simulink model "CoP"  (R2014a)
settings: Solver=ode45  StartTime=0.0  StopTime=10.0  RelTol=1e-3
values from neighbouring files (symbols this model uses):
  l_ankle_pitch = 18    [parameters.m]
  l_ankle_roll = 19    [parameters.m]
libraries: WBCLibrary x6
settings Model: Creator=luca  LastModifiedBy=luca

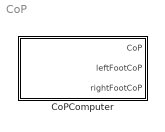
== system CoP ==
  CoPComputer : Subsystem

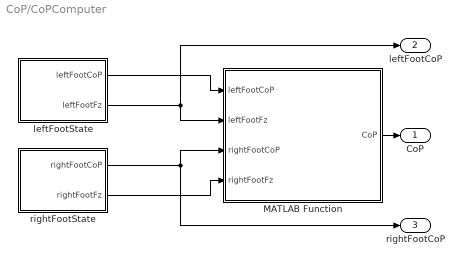
== system CoP/CoPComputer ==
  MATLAB Function : MATLAB Function  TreatAsAtomicUnit=on
  leftFootState : Subsystem
  rightFootState : Subsystem
  CoP : Outport
  leftFootCoP : Outport  Port=2
  rightFootCoP : Outport  Port=3
  wires:
  rightFootState/1(rightFootCoP) -> rightFootCoP/1, MATLAB Function/3(rightFootCoP)
  leftFootState/1(leftFootCoP) -> MATLAB Function/1(leftFootCoP)
  leftFootState/2(leftFootFz) -> leftFootCoP/1, MATLAB Function/2(leftFootFz)
  rightFootState/2(rightFootFz) -> MATLAB Function/4(rightFootFz)
  MATLAB Function/1(CoP) -> CoP/1

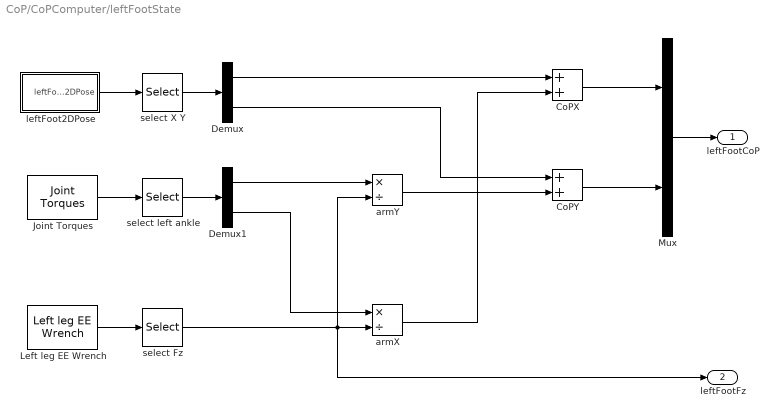
== system CoP/CoPComputer/leftFootState ==
  CoPX : Sum
  CoPY : Sum
  Demux : Demux  Outputs=2
  Demux1 : Demux  Outputs=2
  Joint Torques : WBCLibrary/wholeBodyStates/Joint Torques  robotName=robotName  localName=localName
  Left leg EE Wrench : WBCLibrary/wholeBodyStates/Left leg EE Wrench  robotName=robotName  localName=localName
  Mux : Mux  Inputs=2
  armX : Product  Inputs=*/
  armY : Product  Inputs=*/
  leftFoot2DPose : Subsystem
  select Fz : Selector  InputPortWidth=25  Indices=[3]
  select X Y : Selector  InputPortWidth=25  Indices=[1, 2]
  select left ankle : Selector  InputPortWidth=25  Indices=[l_ankle_pitch, l_ankle_roll]
  leftFootCoP : Outport
  leftFootFz : Outport  Port=2
  wires:
  Left leg EE Wrench/1 -> select Fz/1
  select left ankle/1 -> Demux1/1
  CoPY/1 -> Mux/2
  CoPX/1 -> Mux/1
  armY/1 -> CoPY/2
  Mux/1 -> leftFootCoP/1
  Demux1/2 -> armX/1
  Demux/2 -> CoPY/1
  Demux/1 -> CoPX/1
  Joint Torques/1 -> select left ankle/1
  armX/1 -> CoPX/2
  Demux1/1 -> armY/1
  select X Y/1 -> Demux/1
  leftFoot2DPose/1(leftFoot2DPose) -> select X Y/1
  select Fz/1 -> leftFootFz/1, armX/2, armY/2

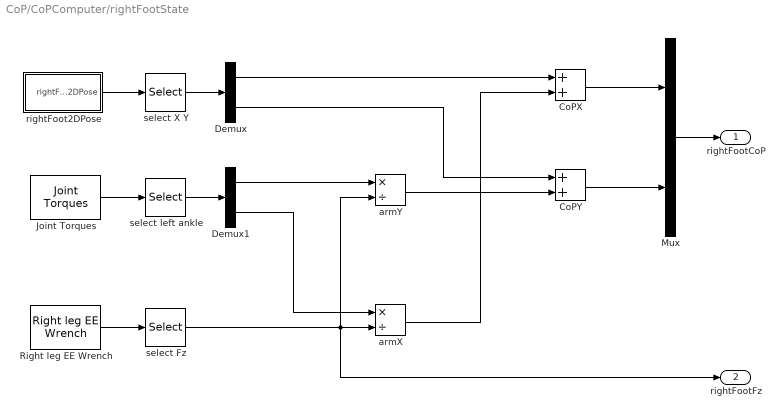
== system CoP/CoPComputer/rightFootState ==
  CoPX : Sum
  CoPY : Sum
  Demux : Demux  Outputs=2
  Demux1 : Demux  Outputs=2
  Joint Torques : WBCLibrary/wholeBodyStates/Joint Torques  robotName=robotName  localName=localName
  Mux : Mux  Inputs=2
  Right leg EE Wrench : WBCLibrary/wholeBodyStates/Right leg EE Wrench  robotName=robotName  localName=localName
  armX : Product  Inputs=*/
  armY : Product  Inputs=*/
  rightFoot2DPose : Subsystem
  select Fz : Selector  InputPortWidth=25  Indices=[3]
  select X Y : Selector  InputPortWidth=25  Indices=[1, 2]
  select left ankle : Selector  InputPortWidth=25  Indices=[l_ankle_pitch, l_ankle_roll]
  rightFootCoP : Outport
  rightFootFz : Outport  Port=2
  wires:
  Right leg EE Wrench/1 -> select Fz/1
  select left ankle/1 -> Demux1/1
  CoPY/1 -> Mux/2
  CoPX/1 -> Mux/1
  armY/1 -> CoPY/2
  Mux/1 -> rightFootCoP/1
  Demux1/2 -> armX/1
  Demux/2 -> CoPY/1
  Demux/1 -> CoPX/1
  Joint Torques/1 -> select left ankle/1
  armX/1 -> CoPX/2
  Demux1/1 -> armY/1
  select X Y/1 -> Demux/1
  rightFoot2DPose/1(rightFoot2DPose) -> select X Y/1
  select Fz/1 -> rightFootFz/1, armX/2, armY/2

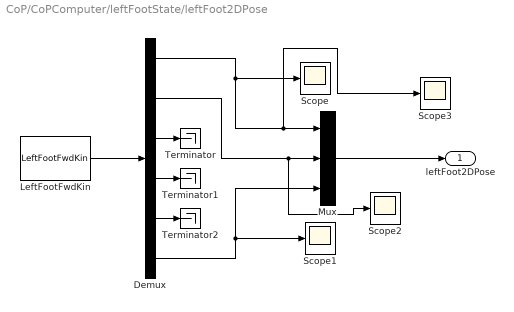
== system CoP/CoPComputer/leftFootState/leftFoot2DPose ==
  Demux : Demux  Outputs=6
  LeftFootFwdKin : WBCLibrary/wholeBodyModel/Forward Kinematics/LeftFootFwdKin  robotName=robotName  localName=localName
      link override Input Param. for forwardKinematics and  computeJacobians 4: Value=zeros(ROBOT_DOF+6,1)
  Mux : Mux  Inputs=3
  Scope{,1..3} (4 alike) : Scope
      Scope1 settings: SaveName=ScopeData2
      Scope2 settings: SaveName=ScopeData3
      Scope3 settings: SaveName=ScopeData4
  Terminator : Terminator
  Terminator1 : Terminator
  Terminator2 : Terminator
  leftFoot2DPose : Outport
  wires:
  Demux/3 -> Terminator/1
  Demux/2 -> Scope2/1, Mux/2
  LeftFootFwdKin/1 -> Demux/1
  Demux/4 -> Terminator1/1
  Demux/5 -> Terminator2/1
  Mux/1 -> leftFoot2DPose/1
  Demux/6 -> Mux/3, Scope1/1
  Demux/1 -> Scope/1, Scope3/1, Mux/1

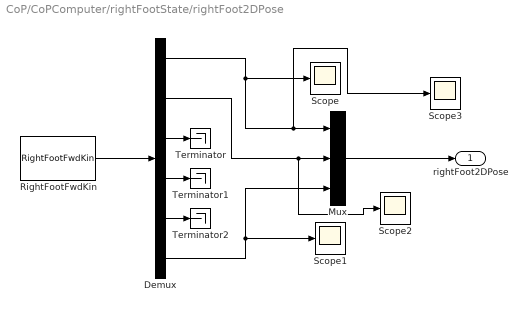
== system CoP/CoPComputer/rightFootState/rightFoot2DPose ==
  Demux : Demux  Outputs=6
  Mux : Mux  Inputs=3
  RightFootFwdKin : WBCLibrary/wholeBodyModel/Forward Kinematics/RightFootFwdKin  robotName=robotName  localName=localName
  Scope{,1..3} (4 alike) : Scope
      Scope1 settings: SaveName=ScopeData2
      Scope2 settings: SaveName=ScopeData3
      Scope3 settings: SaveName=ScopeData4
  Terminator : Terminator
  Terminator1 : Terminator
  Terminator2 : Terminator
  rightFoot2DPose : Outport
  wires:
  Demux/3 -> Terminator/1
  Demux/2 -> Scope2/1, Mux/2
  RightFootFwdKin/1 -> Demux/1
  Demux/4 -> Terminator1/1
  Demux/5 -> Terminator2/1
  Mux/1 -> rightFoot2DPose/1
  Demux/6 -> Mux/3, Scope1/1
  Demux/1 -> Scope/1, Scope3/1, Mux/1

== matlab function CoP/CoPComputer/MATLAB Function ==
  data: leftFootCoP input; leftFootFz input; CoP output; rightFootCoP input; rightFootFz input
function CoP = fcn(leftFootCoP, leftFootFz, rightFootCoP, rightFootFz)
leftFootCoPX = leftFootCoP(1);
leftFootCoPY = leftFootCoP(2);
rightFootCoPX = rightFootCoP(1);
rightFootCoPY = rightFootCoP(2);
totFz = leftFootFz + rightFootFz;

CoPX = (leftFootCoPX * leftFootFz + rightFootCoPX * rightFootFz) / totFz; 
CoPY = (leftFootCoPY * leftFootFz + rightFootCoPY * rightFootFz) / totFz;

CoP = [CoPX, CoPY];
